simulink model "closedLoop_Harness_Observer"  (R2019a)
settings: Solver=FixedStepAuto  StartTime=0.0  StopTime=20  RelTol=1e-3
libraries: controlLibrary x6
Description:
  | Copyright 2008-2019 The MathWorks, Inc.
  | 
  | Observer model
settings Model: Creator=falderis  LastModifiedBy=falderis

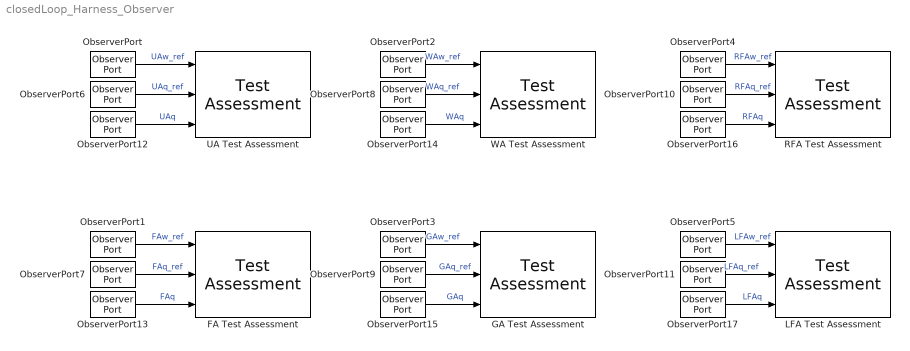
== system closedLoop_Harness_Observer ==
  FA Test Assessment : controlLibrary/Test Assessment  Tag=__SLT_ASMT__  SystemSampleTime=-1
  GA Test Assessment : controlLibrary/Test Assessment  Tag=__SLT_ASMT__  SystemSampleTime=-1
  LFA Test Assessment : controlLibrary/Test Assessment  Tag=__SLT_ASMT__  SystemSampleTime=-1
  ObserverPort{,1..17} (18 alike) : ObserverPort
  RFA Test Assessment : controlLibrary/Test Assessment  Tag=__SLT_ASMT__  SystemSampleTime=-1
  UA Test Assessment : controlLibrary/Test Assessment  Tag=__SLT_ASMT__  SystemSampleTime=-1
  WA Test Assessment : controlLibrary/Test Assessment  Tag=__SLT_ASMT__  SystemSampleTime=-1
  wires:
  ObserverPort/1 -> UA Test Assessment/1  "UAw_ref"
  ObserverPort1/1 -> FA Test Assessment/1  "FAw_ref"
  ObserverPort2/1 -> WA Test Assessment/1  "WAw_ref"
  ObserverPort3/1 -> GA Test Assessment/1  "GAw_ref"
  ObserverPort4/1 -> RFA Test Assessment/1  "RFAw_ref"
  ObserverPort5/1 -> LFA Test Assessment/1  "LFAw_ref"
  ObserverPort6/1 -> UA Test Assessment/2  "UAq_ref"
  ObserverPort7/1 -> FA Test Assessment/2  "FAq_ref"
  ObserverPort8/1 -> WA Test Assessment/2  "WAq_ref"
  ObserverPort9/1 -> GA Test Assessment/2  "GAq_ref"
  ObserverPort10/1 -> RFA Test Assessment/2  "RFAq_ref"
  ObserverPort11/1 -> LFA Test Assessment/2  "LFAq_ref"
  ObserverPort12/1 -> UA Test Assessment/3  "UAq"
  ObserverPort13/1 -> FA Test Assessment/3  "FAq"
  ObserverPort14/1 -> WA Test Assessment/3  "WAq"
  ObserverPort15/1 -> GA Test Assessment/3  "GAq"
  ObserverPort16/1 -> RFA Test Assessment/3  "RFAq"
  ObserverPort17/1 -> LFA Test Assessment/3  "LFAq"
